simulink model "MM1"  (R2019b)
settings: Solver=VariableStepDiscrete  StartTime=0.0  StopTime=stopTime  FixedStep=0.01  RelTol=1e-3
undefined symbols (not defined in the file or in its folder): m, n
settings Model: Creator=pcuijper  LastModifiedBy=pcuijper
settings SolverCC: ZeroCrossControl=DisableAll
settings DataIOCC: ReturnWorkspaceOutputs=off
settings DebuggingCC: ArithmeticOperatorsInVariantConditions=warning
settings SFSimCC: SimUseLocalCustomCode=off  CustomCodeUndefinedFunction=UseInterfaceOnly
settings RTWCC: RTWUseLocalCustomCode=off
settings CodeAppCC: StateflowObjectComments=on

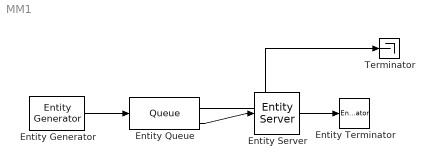
== system MM1 ==
  Entity Generator : EntityGenerator  OutputPortMessageModes=m  TimeSource=MATLAB action  IntergenerationTimeAction=|  GenerateEntityAtSimulationStart=off  EntityType=Structured  EntityTypeName=Entity
      | persistent rngInit;
      | 
      | if isempty(rngInit)
      |     seed = mySeed;
      |     rng(seed);
      |     rngInit = true;
      | end
      | 
      | dt = -interArrivalTime * log(1 - rand());
  Entity Queue : Queue  InputPortMessageModes=m  OutputPortMessageModes=n,m  Capacity=inf  NumberEntitiesInBlock=on
      settings: OutputPortMap=o1,o5
  Entity Server : EntityServer  InputPortMessageModes=m  OutputPortMessageModes=m  Capacity=1  ServiceTimeSource=MATLAB action  ServiceTimeValue=rand(1,1)  ServiceTimeAction=|
      | persistent rngInit;
      | 
      | if isempty(rngInit)
      |     seed = mySeed+1;
      |     rng(seed);
      |     rngInit = true;
      | end
      | 
      | dt = -interServiceTime * log(1 - rand());
  Entity Terminator : EntityTerminator  InputPortMessageModes=m
  Terminator : Terminator
  wires:
  Entity Generator/1 -> Entity Queue/1
  Entity Queue/2 -> Entity Server/1
  Entity Server/1 -> Entity Terminator/1
  Entity Queue/1 -> Terminator/1
